simulink model "Controlador_ON_OFF"  (R2026a)
settings: Solver=VariableStepAuto
values from neighbouring files (symbols this model uses):
  den_planta = [tau 1]    [Controlador_ON_OFF_COD.m]
  histeresis_inf = -0.5    [Controlador_ON_OFF_COD.m]
  histeresis_sup = 0.5    [Controlador_ON_OFF_COD.m]
  num_planta = [K]    [Controlador_ON_OFF_COD.m]
  t_step = 1    [Controlador_ON_OFF_COD.m]
settings Model: Creator=Nehir RT  LastModifiedBy=Nehir RT

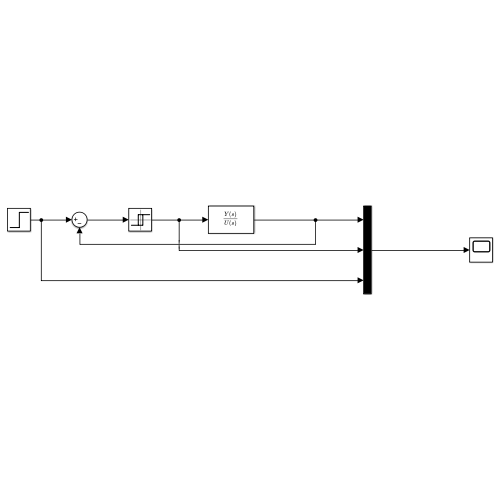
[thumbnail: Simulink's stored preview of the top-level diagram]
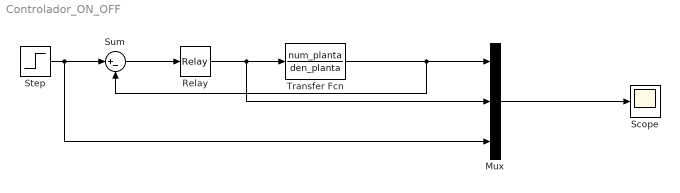
== system Controlador_ON_OFF ==
  Mux : Mux  Inputs=3
  Relay : Relay  OnSwitchValue=histeresis_sup  OffSwitchValue=histeresis_inf  OnOutputValue=out_ON  OffOutputValue=out_OFF
  Scope : Scope
      settings: ActiveDisplayYMinimum=-71.099187960021737  ActiveDisplayYMaximum=108.60096790983486
  Step : Step  Time=t_step  InitialValue=SP_ini  FinalValue=SP_fin  SampleTime=0
  Sum : Sum  Inputs=|+-
  Transfer Fcn : TransferFcn  Numerator=num_planta  Denominator=den_planta
  wires:
  Step/1 -> Mux/3, Sum/1
  Sum/1 -> Relay/1
  Relay/1 -> Mux/2, Transfer Fcn/1
  Transfer Fcn/1 -> Sum/2, Mux/1
  Mux/1 -> Scope/1
